simulink model "LoneWolfSimulator"  (R2023b)
settings: Solver=VariableStepAuto  StartTime=0.0  StopTime=Inf  FixedStep=0.0001  RelTol=1e-6  AbsTol=1e-6
model workspace (MAT data in the model file):
  SL_ROS_VariableLengthArrays_MaxSizes.CommonInfo.ArrayTruncateAction = 'EmitWarning'
  SL_ROS_VariableLengthArrays_MaxSizes.MsgTypeMap = containers.Map
  SL_ROS_VariableLengthArrays_MaxSizes.MsgTypeMap.serialization.keys = {'std_msgs/Float64MultiArray'}
  SL_ROS_VariableLengthArrays_MaxSizes.MsgTypeMap.serialization.values{1}.PropertyName = 'data'
  SL_ROS_VariableLengthArrays_MaxSizes.MsgTypeMap.serialization.values{1}.DataType = 'double'
  SL_ROS_VariableLengthArrays_MaxSizes.MsgTypeMap.serialization.values{1}.MaxLength = 781
  SL_ROS_VariableLengthArrays_MaxSizes.MsgTypeMap.serialization.uniformity = 0
  SL_ROS_VariableLengthArrays_MaxSizes.MsgTypeMap.serialization.keyType = 'char'
  SL_ROS_VariableLengthArrays_MaxSizes.MsgTypeMap.serialization.valueType = 'any'
values from neighbouring files (symbols this model uses):
  alpha_peak = 0.18    [LoneWolfParams.m]
  Bc = 10    [LoneWolfParams.m]
  Bl = 10    [LoneWolfParams.m]
  Cc = 1.9    [LoneWolfParams.m]
  Cl = 1.9    [LoneWolfParams.m]
  Dc = 1*g*m/2    (= 1839.375)    [LoneWolfParams.m]
  Dl = 1*g*m/2    (= 1839.375)    [LoneWolfParams.m]
  Ec = 0.97    [LoneWolfParams.m]
  El = 0.97    [LoneWolfParams.m]
  Iw = 0.5    [LoneWolfParams.m]
  Iz = (1/12) * m * (width^2 + len^2)    (= 225.015625)    [LoneWolfParams.m]
  kappa_peak = 0.18    [LoneWolfParams.m]
  m = 375    [LoneWolfParams.m]
  RRC = 5    [LoneWolfParams.m]
  wheelRadius = 0.33    [LoneWolfParams.m]
  xdotinit = 1e-3    (= 0.001)    [LoneWolfParams.m]
undefined symbols (not defined in the file or in its folder): latitude, longitude
libraries: ros2lib x11, sldrtlib x1
settings Model: Creator=bakke  LastModifiedBy=lonewolf
settings SolverCC: AutoScaleAbsTol=off  EnableFixedStepZeroCrossing=on  MaxZcBracketingIterations=100
settings OptimizationCC: EnhancedBackFolding=on  PassReuseOutputArgsAs=Individual arguments  ZeroExternalMemoryAtStartup=off  ZeroInternalMemoryAtStartup=off  MaxStackSize=64  OptimizeBlockOrder=speed  DifferentSizesBufferReuse=on  EfficientTunableParamExpr=on
settings DebuggingCC: ParameterTunabilityLossMsg=error
settings HardwareCC: ProdBitPerLong=64  ProdHWDeviceType=Intel->x86-64 (Linux 64)  UseEmbeddedCoderFeatures=off
settings RTWCC: Description=Embedded Coder  SystemTargetFile=ert.tlc  HardwareBoard=Robot Operating System 2 (ROS 2)  TLCOptions="-aInlineSetEventsForThisBaseRateFcn=TLC_FALSE -aSuppressMultiTaskScheduler=TLC_FALSE  -aRateBasedStepFcn=0"  TemplateMakefile=ert_default_tmf  Toolchain=Colcon Tools  TargetLang=C++
settings CodeAppCC: ForceParamTrailComments=on  IgnoreCustomStorageClasses=off  OperatorAnnotations=on  SimulinkDataObjDesc=on  SFDataObjDesc=on  InsertBlockDesc=on
settings ERTTargetCC: CodeInterfacePackaging=C++ class  SupportNonInlinedSFcns=on  RootIOFormat=Structure reference

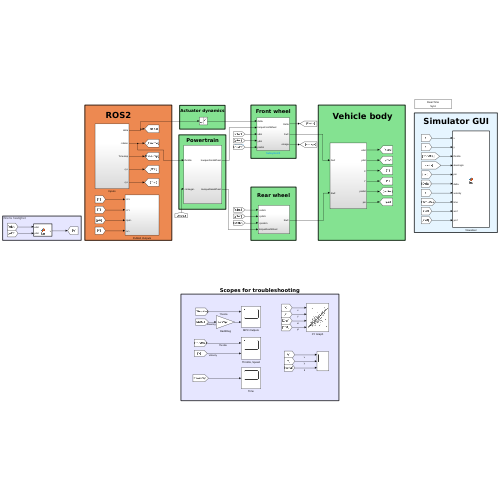
[thumbnail: Simulink's stored preview of the top-level diagram]
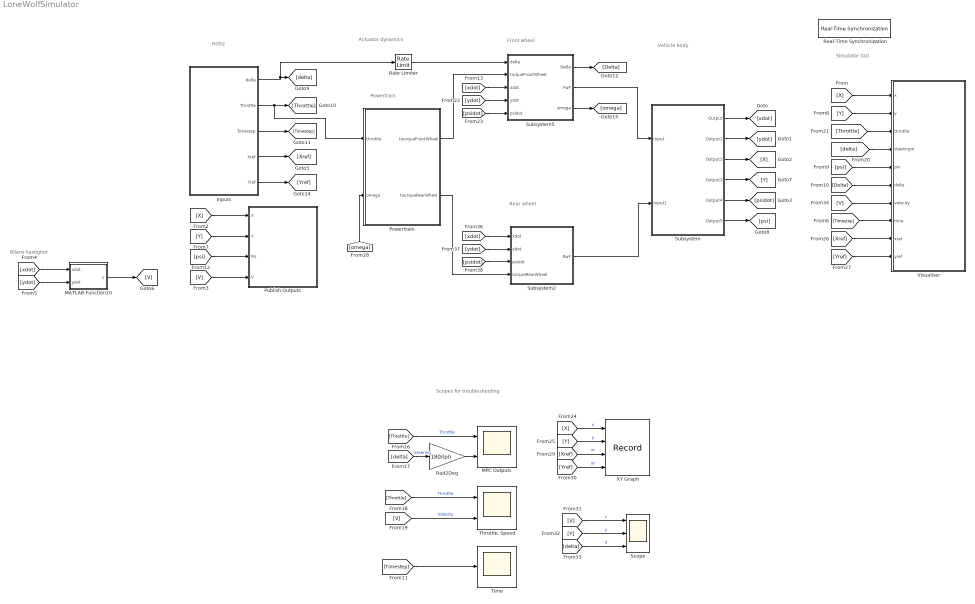
== system LoneWolfSimulator ==
  note: ROS2
  note: Bilens hastighet
  note: Simulator GUI
  note: Vehicle body
  note: Front wheel
  note: Rear wheel
  note: Powertrain
  note: Actuator dynamics
  note: Scopes for troubleshooting
  Inputs : Subsystem
  MATLAB Function10 : MATLAB Function  TreatAsAtomicUnit=on
  MPC Outputs : Scope  NumInputPorts=2
  Powertrain : Subsystem
  Publish Outputs : Subsystem
  Rad2Deg : Gain  Gain=180/(pi)
  Rate Limiter : RateLimiter  RisingSlewLimit=pi/2  FallingSlewLimit=-pi/2
  Real-Time Synchronization : sldrtlib/Real-Time Synchronization  SampleTime=0.1  MaxMissedTicks=1000  ShowMissedTicks=off  YieldWhenWaiting=off
  Scope : Scope  NumInputPorts=3
  Subsystem : Subsystem
  Subsystem2 : Subsystem
  Subsystem5 : Subsystem
  "Throttle, Speed" : Scope  NumInputPorts=2
  Time : Scope
  Visualiser : MATLAB Function  TreatAsAtomicUnit=on
  XY Graph : Record  FileSettingsInternal="{\"entries\":[{\"content\":{\"excelSettings\":{\"content\":{},\"type\":\"Streamout.ExcelSettings\"}},\"type\":\"Streamout.FileSettingStorage\",\"uuid\":\"\"}],\"packageUris\":[\"http:\\/\\/schema.mathworks.com\\/mf0\\/streamout_blocks\\/R2020a\"],\"version\":\"1.0\"}"  Layout=[1 1]  SignalsInternal="{\"entries\":[{\"content\":{\"signals\":[{\"content\":{\"blockPath\":[],\"dimensions\":[1],\"domain\":\"\",\"lineColor\":\"#edb120\",\"plots\":[ 1 ],\"port\":1,\"sid\":[\"\"],\"signalID\":1,\"signalName\":\"x\"},\"type\":\"RecordBlkView.Signal\",\"uuid\":\"\"},{\"content\":{\"blockPath\":[],\"dimensions\":[1],\"domain\":\"\",\"lineColor\":\"#7e2f8e\",\"plots\":[ 1 ],\"port\":2,\"sid\":[\"\"],\"signalID\":2,\"signalName\":\"y\"},\"type\":\"RecordBlkView.Signal\",\"uuid\":\"\"},{\"content\":{\"blockPath\":[],\"dimensions\":[1],\"domain\":\"\",\"lineColor\":\"#77ac30\",\"plots\":[ 1 ],\"port\":3,\"sid\":[\"\"],\"signalID\":3,\"signalName\":\"xr\"},\"type\":\"RecordBlkView.Signal\",\"uuid\":\"\"},{\"content\":{\"blockPath\":[],\"dimensions\":[1],\"domain\":\"\",\"lineColor\":\"#4dbeee\",\"plots\":[ 1 ],\"port\":4,\"sid\":[\"\"],\"signalID\":4,\"signalName\":\"yr\"},\"type\":\"RecordBlkView.Signal\",\"uuid\":\"\"}]},\"type\":\"RecordBlkView.InputSignals\",\"uuid\":\"\"}],\"packageUris\":[\"http:\\/\\/schema.mathworks.com\\/mf0\\/streamout_blocks\\/R2020a\"],\"version\":\"1.0\"}"  VisualizationBindings="{\"xyplotplugin\":{\"info\":[{\"series\":[{\"bindingParametersList\":[{\"parameter\":\"X-Axis\",\"signalID\":1,\"signalName\":\"x\"},{\"parameter\":\"Y-Axis\",\"signalID\":2,\"signalName\":\"y\"}],\"seriesID\":0},{\"bindingParametersList\":[{\"parameter\":\"X-Axis\",\"signalID\":3,\"signalName\":\"xr\"},{\"parameter\":\"Y-Axis\",\"signalID\":4,\"signalName\":\"yr\"}],\"seriesID\":1}],\"subplotID\":1}]}}"  CompatibilityTag=XY
  wires:
  MATLAB Function10/1(v) -> [V]
  [ydot] -> MATLAB Function10/2(ydot)
  Subsystem/1(Output) -> [xdot]
  [xdot] -> MATLAB Function10/1(xdot)
  Subsystem/2(Output1) -> [ydot]
  Subsystem/5(Output4) -> [psidot]
  Subsystem/4(Output3) -> [Y]
  Subsystem/3(Output2) -> [X]
  Subsystem/6(Output5) -> [psi]
  [X] -> Publish Outputs/1(X)
  [Y] -> Publish Outputs/2(Y)
  [psi] -> Publish Outputs/3(Psi)
  [V] -> Publish Outputs/4(V)
  [Throttle] -> MPC Outputs/1  "Throttle"
  [delta] -> Rad2Deg/1  "Steering"
  [Throttle] -> "Throttle, Speed"/1  "Throttle"
  Rad2Deg/1 -> MPC Outputs/2
  Inputs/3(Timestep) -> [Timestep]
  Inputs/4(Xref) -> [Xref]
  Inputs/5(Yref) -> [Yref]
  [omega] -> Powertrain/2(omega)
  [Timestep] -> Time/1
  [V] -> "Throttle, Speed"/2  "Velocity"
  [X] -> XY Graph/1  "x"
  [Y] -> XY Graph/2  "y"
  [Xref] -> XY Graph/3  "xr"
  [Yref] -> XY Graph/4  "yr"
  [V] -> Scope/1  "v"
  [Y] -> Scope/2  "y"
  [delta] -> Scope/3  "d"
  [V] -> Visualiser/7(velocity)
  [Delta] -> Visualiser/6(delta)
  [psi] -> Visualiser/5(psi)
  [delta] -> Visualiser/4(steeringin)
  [Throttle] -> Visualiser/3(throttle)
  [Y] -> Visualiser/2(y)
  [X] -> Visualiser/1(x)
  [Xref] -> Visualiser/9(xref)
  [Timestep] -> Visualiser/8(time)
  [Yref] -> Visualiser/10(yref)
  Powertrain/1(tourqueFrontWheel) -> Subsystem5/2(torqueFrontWheel)
  Subsystem5/1(Delta) -> [Delta]
  Subsystem5/2(FwF) -> Subsystem/1(Input)
  Subsystem5/3(omega) -> [omega]
  Powertrain/2(tourqueRearWheel) -> Subsystem2/4(torqueRearWheel)
  Subsystem2/1(RwF) -> Subsystem/2(Input1)
  Inputs/1(delta) -> [delta], Rate Limiter/1
  Inputs/2(Throttle) -> Powertrain/1(throttle), [Throttle]
  [xdot] -> Subsystem5/3(xdot)
  [ydot] -> Subsystem5/4(ydot)
  [psidot] -> Subsystem5/5(psidot)
  [xdot] -> Subsystem2/1(xdot)
  [ydot] -> Subsystem2/2(ydot)
  [psidot] -> Subsystem2/3(psidot)
  Rate Limiter/1 -> Subsystem5/1(delta)

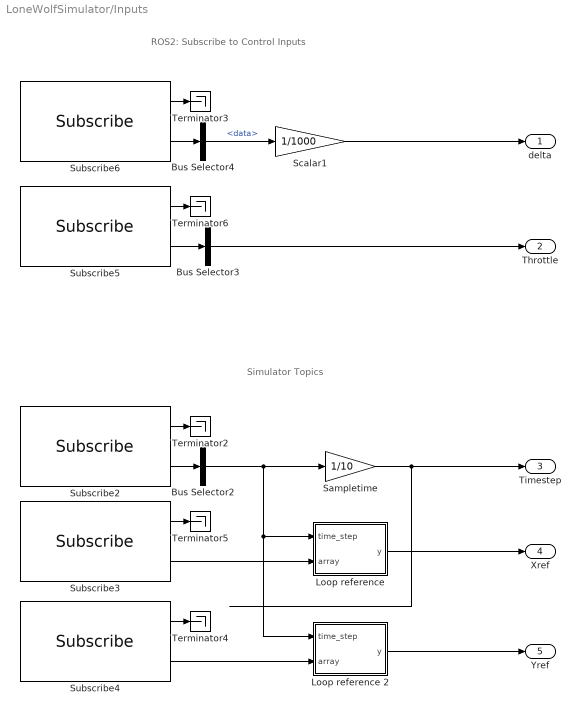
== system LoneWolfSimulator/Inputs ==
  note: ROS2: Subscribe to Control Inputs
  note: Simulator Topics
  Bus Selector2 : BusSelector  OutputSignals=data  OutputAsBus=on
  Bus Selector3 : BusSelector  OutputSignals=data  OutputAsBus=on
  Bus Selector4 : BusSelector  OutputSignals=data
  Loop reference : MATLAB Function  TreatAsAtomicUnit=on
  "Loop reference 2 " : MATLAB Function  TreatAsAtomicUnit=on
  Sampletime : Gain  Gain=1/10
  Scalar1 : Gain  Gain=1/1000
  Subscribe2 : ros2lib/Subscribe  topicSource=Specify your own  topic=/timestep  messageType=std_msgs/Int64  sampleTime=0.1  QOSHistory=Keep last  QOSDepth=1  QOSReliability=Reliable  QOSDurability=Volatile
  Subscribe3 : ros2lib/Subscribe  topicSource=Specify your own  topic=/xref  messageType=std_msgs/Float64MultiArray  sampleTime=0.1  QOSHistory=Keep last  QOSDepth=1  QOSReliability=Reliable  QOSDurability=Volatile
  Subscribe4 : ros2lib/Subscribe  topicSource=Specify your own  topic=/yref  messageType=std_msgs/Float64MultiArray  sampleTime=0.1  QOSHistory=Keep last  QOSDepth=1  QOSReliability=Reliable  QOSDurability=Volatile
  Subscribe5 : ros2lib/Subscribe  topicSource=Specify your own  topic=/lw_portenta_throttle  messageType=std_msgs/Int64  sampleTime=0.1  QOSHistory=Keep last  QOSDepth=1  QOSReliability=Reliable  QOSDurability=Volatile
  Subscribe6 : ros2lib/Subscribe  topicSource=Specify your own  topic=/lw_portenta_steering  messageType=std_msgs/Int64  sampleTime=0.1  QOSHistory=Keep last  QOSDepth=1  QOSReliability=Reliable  QOSDurability=Volatile
  Terminator{2..6} (5 alike) : Terminator
  delta : Outport
  Throttle : Outport  Port=2
  Timestep : Outport  Port=3
  Xref : Outport  Port=4
  Yref : Outport  Port=5
  wires:
  Subscribe2/1 -> Terminator2/1
  Subscribe2/2 -> Bus Selector2/1
  Sampletime/1 -> Timestep/1
  Subscribe4/1 -> Terminator4/1
  Subscribe4/2 -> "Loop reference 2 "/2(array)
  Subscribe3/2 -> Loop reference/2(array)
  Subscribe3/1 -> Terminator5/1
  Loop reference/1(y) -> Xref/1
  "Loop reference 2 "/1(y) -> Yref/1
  Bus Selector2/1 -> Sampletime/1, "Loop reference 2 "/1(time_step), Loop reference/1(time_step)
  Subscribe5/2 -> Bus Selector3/1
  Scalar1/1 -> delta/1
  Bus Selector3/1 -> Throttle/1
  Subscribe6/1 -> Terminator3/1
  Subscribe5/1 -> Terminator6/1
  Subscribe6/2 -> Bus Selector4/1
  Bus Selector4/1 -> Scalar1/1  "<data>"

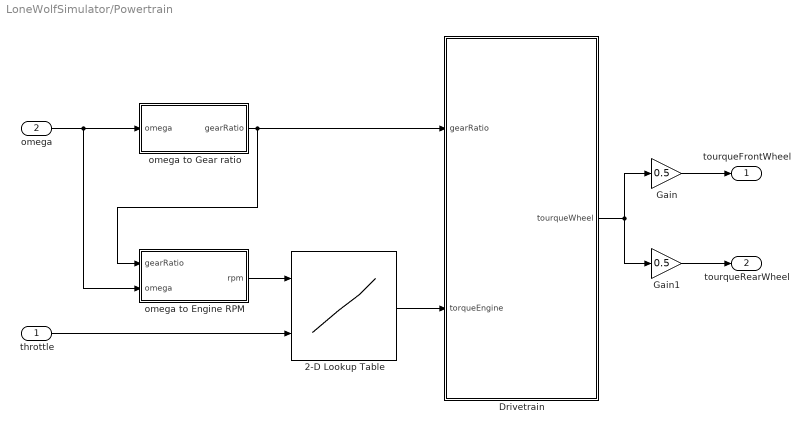
== system LoneWolfSimulator/Powertrain ==
  throttle : Inport
  omega : Inport  Port=2
  2-D Lookup Table : Lookup_n-D  BreakpointsForDimension1=[0;169.614855264094;367.085957899886;589.246670617181;789.821522752712;996.567251474744;1181.71186027627;1425.48895225281;1626.06685625609;1835.92854194885;2042.68342627413;2243.26743401291;2425.36017506641;2616.68481605769;2860.48021924071;3085.77825200297;3264.76724355674;3468.45194892751;3656.70641096427;3909.77338836579;4131.97377536381;4314.05736081407;4493.04635236784;4696.71885026762;4909.65376678264;5110.24998199241;5292.32135997168;5499.07014056146;5718.17288179523;5965.03541206502;6199.56534476505;6390.87472641759;6582.16884873138;6758.05409078541;6980.20259603171]  BreakpointsForDimension2=[0;10;20;30;40;50;60;70;80;90;100]  Table=[0.3 7.52683562951347 11.8387627553835 13.7538912505429 14.2370681748395 17.110514311951 18.5474885119643 17.5896731329271 18.0683296909882 19.0271495958556 24.298398889508;0.2 10.3686392029757 12.7749808290727 17.5615464096832 19.4852133743988 21.8820120051095 25.2300965969615 24.7539513534759 28.0985201049223 31.4546409034155 33.8484259566359;0 11.2978255958539 15.1431504736246 22.3255101591157 25.2084992916136 29.038254019017 37.6505562237105 34.7881598707304 46.2688855833847 47.2272032253369 51.5386280882919;0 13.1858318935994 20.8624182875188 30.4380607633152 37.1492978344714 39.5491100426724 54.8631063231358 53.915838465315 65.4061071733557 67.8013990153211 73.0706392573133;0 16.0346671478725 30.4094317771563 43.3462176805965 52.4527465937181 63.4723949503387 69.6994505713682 77.3680007586463 84.553876284543 88.8678124620733 88.8688169879034;-2.44629412790408 24.6344127796893 47.1563841543122 73.0294536982776 73.0379921678338 91.720665819667 102.743327753778 118.552053005585 116.160277004025 127.660088707451 124.308990538109;-4.96800884998436 35.1502914324955 71.0816781136389 103.177785175313 114.222546677687 132.430079611865 148.722986313798 180.336920977006 188.48362545943 193.279734035427 163.107293938468;-8.74578514092923 33.6856927721534 72.4880142758329 104.587637177913 130.961462848202 155.87470796147 177.437859431226 195.635347107102 209.529446126664 221.029760093006 226.319090851601;-12.1015317204333 33.6520411568438 75.3288133234649 113.858360154898 143.370370427905 164.462399283325 190.810609544946 214.287382721116 229.13779033097 243.993220569975 247.83502960734;-19.201920026761 35.0558660044625 81.0551128181702 121.980453754484 158.198176206581 185.034586021649 211.865973207567 232.947956804686 250.676330917887 265.053104598831 277.032075123234;-23.3903905203684 35.0282415441337 84.3810978417591 127.227594428213 165.359943112554 196.510289105152 225.735461344291 249.691393341436 267.899930801444 284.190326188802 296.649460060012;-27.5779890517621 31.4144554912304 86.2680996136746 133.424012011423 173.479023134649 206.067347853091 234.811352219593 263.073686450543 283.200365983201 296.143179041622 314.343680294988;-34.6744535281279 28.5083622646395 84.8029986904173 132.424508810435 174.403689161292 210.348636941142 239.083600575173 265.9119741836 288.438465924458 303.782095716911 318.144303773318;-38.4448181402563 22.7303296896822 79.0219525379695 127.60881198075 170.065644363838 207.922707061357 236.655159380812 261.571418071571 285.059241031872 302.791633248394 315.243735438792;-44.7181502868699 19.3501002712657 76.5965249210998 125.188909255946 170.034504063104 205.489745500762 237.114227685186 262.989306280812 284.552457750567 303.239651768636 317.613914135005;-53.0684964265662 14.5328966528359 72.7336208413018 123.725817384349 168.093257896361 204.501292083905 235.646615447353 263.444356481864 285.961807490252 304.168335898599 318.061932655246;-57.6689690661566 10.1943495924673 67.9169194857871 119.863917830381 165.197712190987 201.122569454234 232.254331718975 261.012399447099 284.010516065207 301.740396967154 318.513467015894;-63.9366334583809 4.41481022876471 62.1353710704242 114.762859997277 162.775298151607 195.485378400082 228.870586460153 255.707498538137 277.747799777208 296.440518687343 312.256777882875;-69.7861919691262 -2.32304677689018 58.7496167599421 109.939629223867 157.474917608881 193.058946257382 225.968009073968 255.203226571407 278.19581829745 296.410885175354 312.707307717692;-78.1404619387842 -9.54508523267177 53.452249794706 105.592543693942 154.556770072328 190.157373397027 224.031785536375 252.782821583688 275.782444990542 295.429463439308 311.718854300836;-84.8266681935945 -12.4471603559423 48.6390642795968 102.692979885247 151.179554231402 188.687752107534 223.0493592745 251.318725186261 274.317344067285 293.481687854669 309.292422158136;-90.6753547421262 -16.3085576469951 45.7379936821564 99.7888957103159 147.799324812986 188.655607280969 222.54508730777 250.807923801635 ...(+2434 chars)]  InternalRulePriority=Speed  RndMeth=Simplest
      settings: InputPortMap=u0,u1
  Drivetrain : MATLAB Function  TreatAsAtomicUnit=on
  Gain : Gain  Gain=0.5
  Gain1 : Gain  Gain=0.5
  omega to Engine RPM : MATLAB Function  TreatAsAtomicUnit=on
  omega to Gear ratio : MATLAB Function  TreatAsAtomicUnit=on
  tourqueFrontWheel : Outport
  tourqueRearWheel : Outport  Port=2
  wires:
  omega to Gear ratio/1(gearRatio) -> omega to Engine RPM/1(gearRatio), Drivetrain/1(gearRatio)
  2-D Lookup Table/1 -> Drivetrain/2(torqueEngine)
  throttle/1 -> 2-D Lookup Table/2
  omega/1 -> omega to Gear ratio/1(omega), omega to Engine RPM/2(omega)
  omega to Engine RPM/1(rpm) -> 2-D Lookup Table/1
  Drivetrain/1(tourqueWheel) -> Gain1/1, Gain/1
  Gain/1 -> tourqueFrontWheel/1
  Gain1/1 -> tourqueRearWheel/1

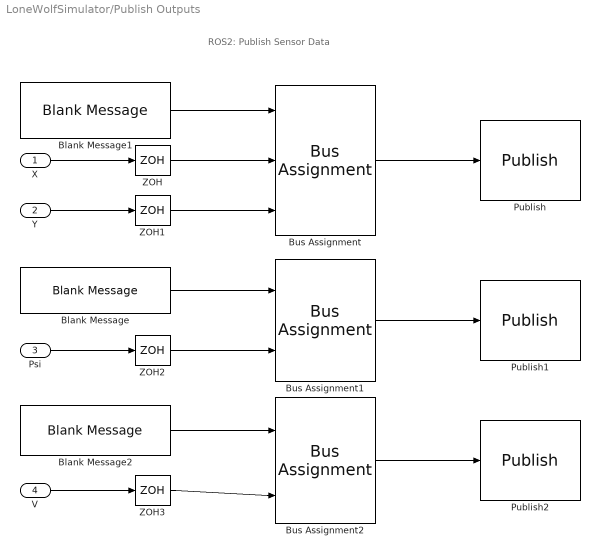
== system LoneWolfSimulator/Publish Outputs ==
  note: ROS2: Publish Sensor Data
  X : Inport
  Y : Inport  Port=2
  Psi : Inport  Port=3
  V : Inport  Port=4
  Blank Message : ros2lib/Blank Message  messageClass=Message  entityType=geometry_msgs/PoseWithCovarianceStamped  messageType=geometry_msgs/PoseWithCovarianceStamped  SampleTime=0.1
  Blank Message1 : ros2lib/Blank Message  messageClass=Message  entityType=sensor_msgs/NavSatFix  messageType=sensor_msgs/NavSatFix  SampleTime=0.1
  Blank Message2 : ros2lib/Blank Message  messageClass=Message  entityType=geometry_msgs/TwistWithCovarianceStamped  messageType=geometry_msgs/TwistWithCovarianceStamped  SampleTime=0.1
  Bus Assignment : BusAssignment  AssignedSignals=latitude,longitude
  Bus Assignment1 : BusAssignment  AssignedSignals=pose.pose.position.z
  Bus Assignment2 : BusAssignment  AssignedSignals=twist.twist.linear.x
  Publish : ros2lib/Publish  topicSource=Specify your own  topic=/vectornav/gnss  messageType=sensor_msgs/NavSatFix  QOSHistory=Keep last  QOSDepth=1  QOSReliability=Reliable  QOSDurability=Volatile
  Publish1 : ros2lib/Publish  topicSource=Specify your own  topic=/vectornav/pose  messageType=geometry_msgs/PoseWithCovarianceStamped  QOSHistory=Keep last  QOSDepth=1  QOSReliability=Reliable  QOSDurability=Volatile
  Publish2 : ros2lib/Publish  topicSource=Specify your own  topic=/vectornav/velocity_body  messageType=geometry_msgs/TwistWithCovarianceStamped  QOSHistory=Keep last  QOSDepth=1  QOSReliability=Reliable  QOSDurability=Volatile
  ZOH{,1..3} (4 alike) : ZeroOrderHold  SampleTime=0.1
  wires:
  Blank Message/1 -> Bus Assignment1/1
  Bus Assignment1/1 -> Publish1/1
  ZOH3/1 -> Bus Assignment2/2
  Bus Assignment2/1 -> Publish2/1
  ZOH2/1 -> Bus Assignment1/2
  Psi/1 -> ZOH2/1
  Blank Message1/1 -> Bus Assignment/1
  V/1 -> ZOH3/1
  X/1 -> ZOH/1
  ZOH/1 -> Bus Assignment/2
  Bus Assignment/1 -> Publish/1
  Blank Message2/1 -> Bus Assignment2/1
  Y/1 -> ZOH1/1
  ZOH1/1 -> Bus Assignment/3

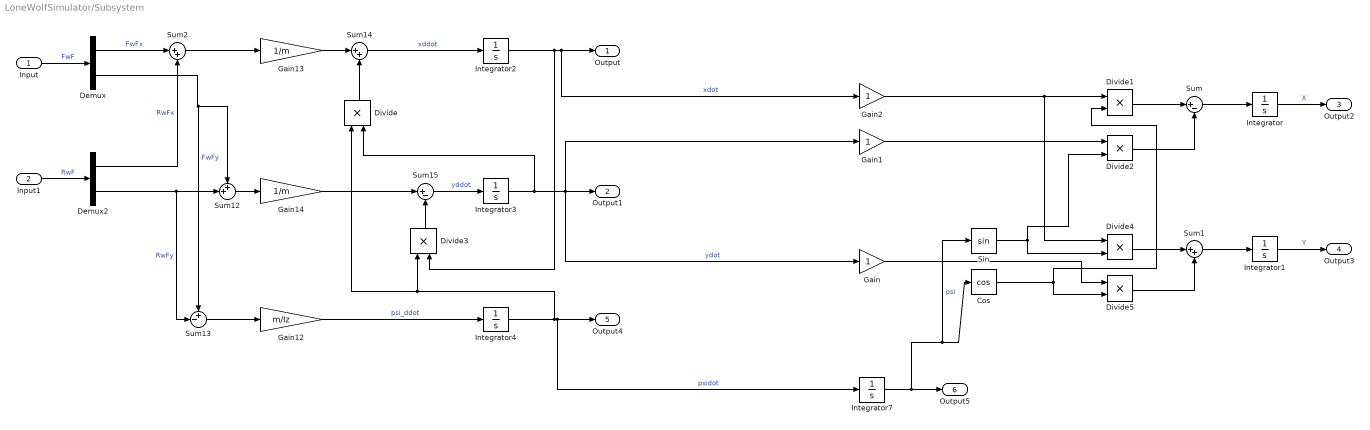
== system LoneWolfSimulator/Subsystem ==
  Input : Inport
  Input1 : Inport  Port=2
  Cos : Trigonometry  Operator=cos
  Demux : Demux  Outputs=2
  Demux2 : Demux  Outputs=2
  Divide{,1..5} (6 alike) : Product  Inputs=**
  Gain : Gain
  Gain1 : Gain
  Gain12 : Gain  Gain=m/Iz
  Gain13 : Gain  Gain=1/m
  Gain14 : Gain  Gain=1/m
  Gain2 : Gain
  Integrator{,1,3..4,7} (5 alike) : Integrator
  Integrator2 : Integrator  InitialCondition=xdotinit
  Sin : Trigonometry
  Sum : Sum  Inputs=|+-
  Sum1 : Sum  Inputs=|++
  Sum12 : Sum  Inputs=++|
  Sum13 : Sum  Inputs=+-|
  Sum14 : Sum  Inputs=|++
  Sum15 : Sum  Inputs=|+-
  Sum2 : Sum  Inputs=|++
  Output : Outport
  Output1 : Outport  Port=2
  Output2 : Outport  Port=3
  Output3 : Outport  Port=4
  Output4 : Outport  Port=5
  Output5 : Outport  Port=6
  wires:
  Demux2/1 -> Sum2/2  "RwFx"
  Input/1 -> Demux/1  "FwF"
  Demux/1 -> Sum2/1  "FwFx"
  Demux2/2 -> Sum12/2, Sum13/2  "RwFy"
  Integrator2/1 -> Gain2/1, Output/1, Divide3/2  "xdot"
  Sum13/1 -> Gain12/1
  Integrator4/1 -> Integrator7/1, Output4/1, Divide/1, Divide3/1  "psidot"
  Sum14/1 -> Integrator2/1  "xddot"
  Demux/2 -> Sum12/1, Sum13/1  "FwFy"
  Input1/1 -> Demux2/1  "RwF"
  Gain13/1 -> Sum14/1
  Integrator7/1 -> Output5/1, Cos/1, Sin/1  "psi"
  Gain14/1 -> Sum15/1
  Integrator3/1 -> Gain1/1, Gain/1, Output1/1, Divide/2  "ydot"
  Divide3/1 -> Sum15/2
  Gain12/1 -> Integrator4/1  "psi_ddot"
  Sum2/1 -> Gain13/1
  Sum15/1 -> Integrator3/1  "yddot"
  Sum12/1 -> Gain14/1
  Divide/1 -> Sum14/2
  Cos/1 -> Divide5/2, Divide1/2
  Sin/1 -> Divide4/2, Divide2/2
  Divide1/1 -> Sum/1
  Divide2/1 -> Sum/2
  Divide4/1 -> Sum1/1
  Divide5/1 -> Sum1/2
  Sum/1 -> Integrator/1
  Integrator/1 -> Output2/1  "X"
  Sum1/1 -> Integrator1/1
  Integrator1/1 -> Output3/1  "Y"
  Gain/1 -> Divide5/1
  Gain1/1 -> Divide2/1
  Gain2/1 -> Divide1/1, Divide4/1

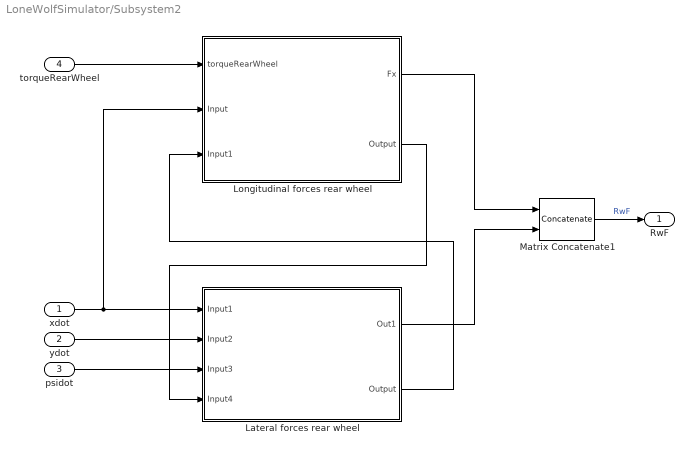
== system LoneWolfSimulator/Subsystem2 ==
  xdot : Inport
  ydot : Inport  Port=2
  psidot : Inport  Port=3
  torqueRearWheel : Inport  Port=4
  Lateral forces rear wheel : Subsystem
  Longitudinal forces rear wheel : Subsystem
  Matrix Concatenate1 : Concatenate  Mode=Multidimensional array
  RwF : Outport
  wires:
  Longitudinal forces rear wheel/2(Output) -> Lateral forces rear wheel/4(Input4)
  Lateral forces rear wheel/2(Output) -> Longitudinal forces rear wheel/3(Input1)
  torqueRearWheel/1 -> Longitudinal forces rear wheel/1(torqueRearWheel)
  xdot/1 -> Lateral forces rear wheel/1(Input1), Longitudinal forces rear wheel/2(Input)
  ydot/1 -> Lateral forces rear wheel/2(Input2)
  psidot/1 -> Lateral forces rear wheel/3(Input3)
  Lateral forces rear wheel/1(Out1) -> Matrix Concatenate1/2
  Longitudinal forces rear wheel/1(Fx) -> Matrix Concatenate1/1
  Matrix Concatenate1/1 -> RwF/1  "RwF"

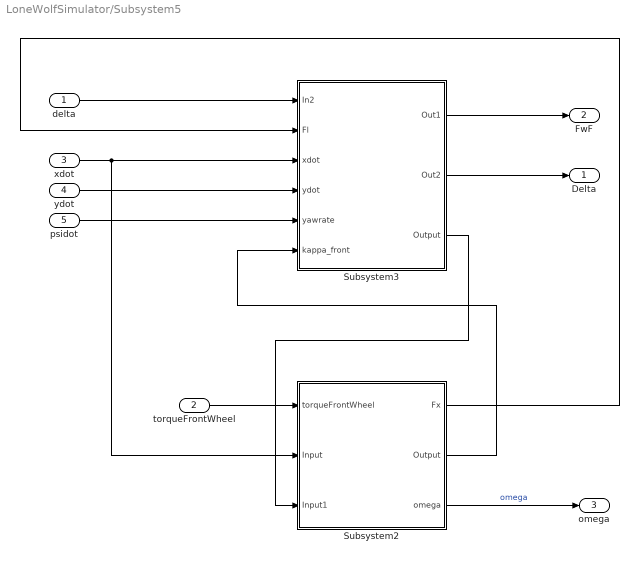
== system LoneWolfSimulator/Subsystem5 ==
  delta : Inport
  torqueFrontWheel : Inport  Port=2
  xdot : Inport  Port=3
  ydot : Inport  Port=4
  psidot : Inport  Port=5
  Subsystem2 : Subsystem
  Subsystem3 : Subsystem
  Delta : Outport
  FwF : Outport  Port=2
  omega : Outport  Port=3
  wires:
  Subsystem2/2(Output) -> Subsystem3/6(kappa_front)
  Subsystem3/2(Out2) -> Delta/1
  Subsystem3/1(Out1) -> FwF/1
  ydot/1 -> Subsystem3/4(ydot)
  psidot/1 -> Subsystem3/5(yawrate)
  Subsystem2/3(omega) -> omega/1  "omega"
  xdot/1 -> Subsystem2/2(Input), Subsystem3/3(xdot)
  torqueFrontWheel/1 -> Subsystem2/1(torqueFrontWheel)
  delta/1 -> Subsystem3/1(In2)
  Subsystem3/3(Output) -> Subsystem2/3(Input1)
  Subsystem2/1(Fx) -> Subsystem3/2(Fl)

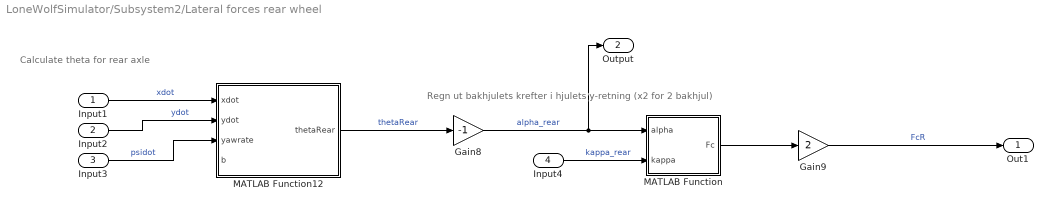
== system LoneWolfSimulator/Subsystem2/Lateral forces rear wheel ==
  note: Regn ut bakhjulets krefter i hjulets y-retning (x2 for 2 bakhjul)
  note: Calculate theta for rear axle
  Input1 : Inport
  Input2 : Inport  Port=2
  Input3 : Inport  Port=3
  Input4 : Inport  Port=4
  Gain8 : Gain  Gain=-1
  Gain9 : Gain  Gain=2
  MATLAB Function : MATLAB Function  TreatAsAtomicUnit=on
  MATLAB Function12 : MATLAB Function  TreatAsAtomicUnit=on
  Out1 : Outport
  Output : Outport  Port=2
  wires:
  Gain9/1 -> Out1/1  "FcR"
  Gain8/1 -> MATLAB Function/1(alpha), Output/1  "alpha_rear"
  MATLAB Function12/1(thetaRear) -> Gain8/1  "thetaRear"
  Input3/1 -> MATLAB Function12/3(yawrate)  "psidot"
  Input2/1 -> MATLAB Function12/2(ydot)  "ydot"
  Input1/1 -> MATLAB Function12/1(xdot)  "xdot"
  MATLAB Function/1(Fc) -> Gain9/1
  Input4/1 -> MATLAB Function/2(kappa)  "kappa_rear"

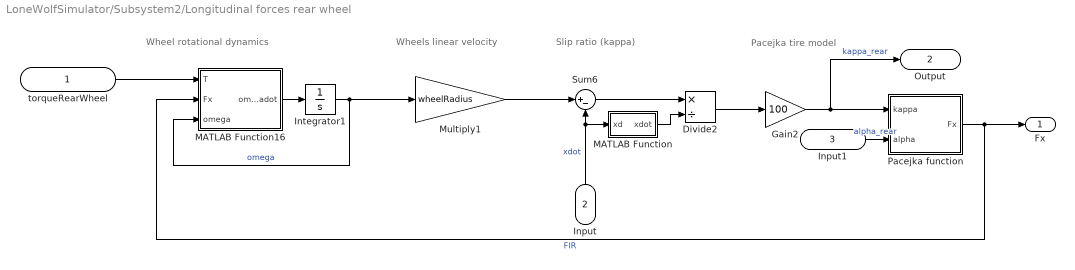
== system LoneWolfSimulator/Subsystem2/Longitudinal forces rear wheel ==
  note: Pacejka tire model
  note: Slip ratio (kappa)
  note: Wheels linear velocity
  note: Wheel rotational dynamics
  torqueRearWheel : Inport
  Input : Inport  Port=2
  Input1 : Inport  Port=3
  Divide2 : Product  Inputs=*/
  Gain2 : Gain  Gain=100
  Integrator1 : Integrator  InitialCondition=(xdotinit)/0.3
  MATLAB Function : MATLAB Function  TreatAsAtomicUnit=on
  MATLAB Function16 : MATLAB Function  TreatAsAtomicUnit=on
  Multiply1 : Gain  Gain=wheelRadius
  Pacejka function : MATLAB Function  TreatAsAtomicUnit=on
  Sum6 : Sum  Inputs=|+-
  Fx : Outport
  Output : Outport  Port=2
  wires:
  Pacejka function/1(Fx) -> Fx/1, MATLAB Function16/2(Fx)  "FlR"
  Divide2/1 -> Gain2/1
  MATLAB Function16/1(omegadot) -> Integrator1/1
  Integrator1/1 -> Multiply1/1, MATLAB Function16/3(omega)  "omega"
  Multiply1/1 -> Sum6/1
  Sum6/1 -> Divide2/1
  Input/1 -> Sum6/2, MATLAB Function/1(xd)  "xdot"
  MATLAB Function/1(xdot) -> Divide2/2
  Gain2/1 -> Pacejka function/1(kappa), Output/1  "kappa_rear"
  torqueRearWheel/1 -> MATLAB Function16/1(T)
  Input1/1 -> Pacejka function/2(alpha)  "alpha_rear"

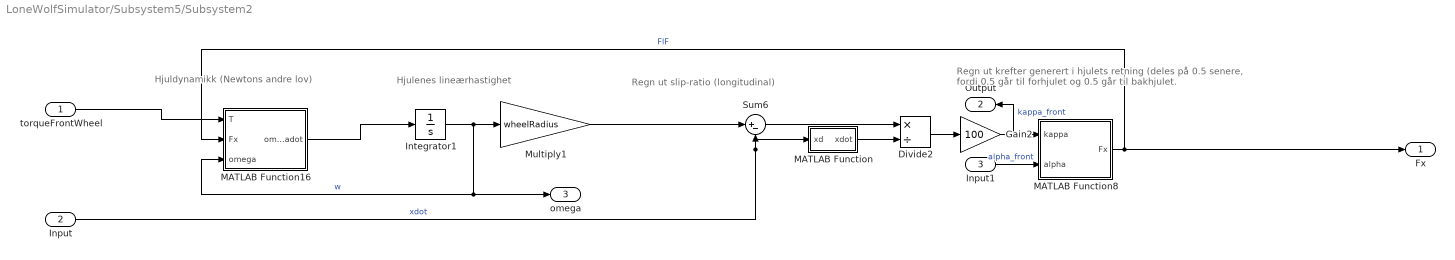
== system LoneWolfSimulator/Subsystem5/Subsystem2 ==
  note: Hjulenes lineærhastighet
  note: Regn ut krefter generert i hjulets retning (deles på 0.5 senere, fordi 0.5 går til forhjulet og 0.5 går til bakhjulet.
  note: Regn ut slip-ratio (longitudinal)
  note: Hjuldynamikk (Newtons andre lov)
  torqueFrontWheel : Inport
  Input : Inport  Port=2
  Input1 : Inport  Port=3
  Divide2 : Product  Inputs=*/
  Gain2 : Gain  Gain=100
  Integrator1 : Integrator  InitialCondition=(xdotinit)/0.3
  MATLAB Function : MATLAB Function  TreatAsAtomicUnit=on
  MATLAB Function16 : MATLAB Function  TreatAsAtomicUnit=on
  MATLAB Function8 : MATLAB Function  TreatAsAtomicUnit=on
  Multiply1 : Gain  Gain=wheelRadius
  Sum6 : Sum  Inputs=|+-
  Fx : Outport
  Output : Outport  Port=2
  omega : Outport  Port=3
  wires:
  MATLAB Function8/1(Fx) -> Fx/1, MATLAB Function16/2(Fx)  "FlF"
  Divide2/1 -> Gain2/1
  MATLAB Function16/1(omegadot) -> Integrator1/1
  Integrator1/1 -> Multiply1/1, omega/1, MATLAB Function16/3(omega)  "w"
  Multiply1/1 -> Sum6/1
  Sum6/1 -> Divide2/1
  Input/1 -> MATLAB Function/1(xd), Sum6/2  "xdot"
  MATLAB Function/1(xdot) -> Divide2/2
  Gain2/1 -> MATLAB Function8/1(kappa), Output/1  "kappa_front"
  torqueFrontWheel/1 -> MATLAB Function16/1(T)
  Input1/1 -> MATLAB Function8/2(alpha)  "alpha_front"

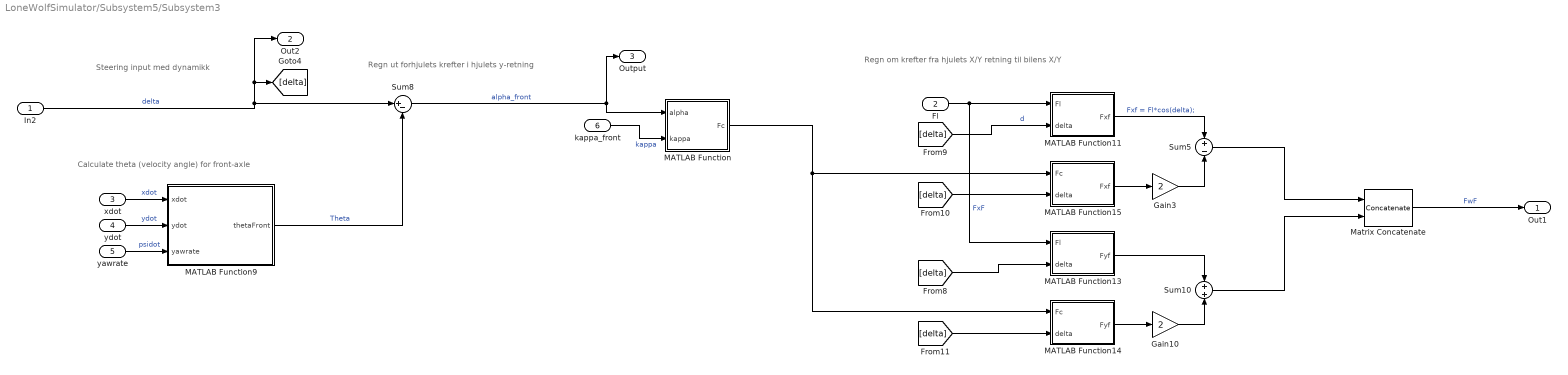
== system LoneWolfSimulator/Subsystem5/Subsystem3 ==
  note: Regn om krefter fra hjulets X/Y retning til bilens X/Y
  note: Steering input med dynamikk
  note: Regn ut forhjulets krefter i hjulets y-retning
  note: Calculate theta (velocity angle) for front-axle
  In2 : Inport
  Fl : Inport  Port=2
  xdot : Inport  Port=3
  ydot : Inport  Port=4
  yawrate : Inport  Port=5
  kappa_front : Inport  Port=6
  Gain10 : Gain  Gain=2
  Gain3 : Gain  Gain=2
  MATLAB Function : MATLAB Function  TreatAsAtomicUnit=on
  MATLAB Function11 : MATLAB Function  TreatAsAtomicUnit=on
  MATLAB Function13 : MATLAB Function  TreatAsAtomicUnit=on
  MATLAB Function14 : MATLAB Function  TreatAsAtomicUnit=on
  MATLAB Function15 : MATLAB Function  TreatAsAtomicUnit=on
  MATLAB Function9 : MATLAB Function  TreatAsAtomicUnit=on
  Matrix Concatenate : Concatenate  Mode=Multidimensional array
  Sum10 : Sum  Inputs=+|+
  Sum5 : Sum  Inputs=+|-
  Sum8 : Sum  Inputs=|+-
  Out1 : Outport
  Out2 : Outport  Port=2
  Output : Outport  Port=3
  wires:
  Gain3/1 -> Sum5/2
  Sum10/1 -> Matrix Concatenate/2
  MATLAB Function11/1(Fxf) -> Sum5/1  "Fxf = Fl*cos(delta);"
  [delta] -> MATLAB Function11/2(delta)  "d"
  MATLAB Function15/1(Fxf) -> Gain3/1
  Sum5/1 -> Matrix Concatenate/1
  [delta] -> MATLAB Function15/2(delta)
  MATLAB Function9/1(thetaFront) -> Sum8/2  "Theta"
  Gain10/1 -> Sum10/2
  [delta] -> MATLAB Function14/2(delta)
  MATLAB Function13/1(Fyf) -> Sum10/1
  Sum8/1 -> Output/1, MATLAB Function/1(alpha)  "alpha_front"
  MATLAB Function14/1(Fyf) -> Gain10/1
  [delta] -> MATLAB Function13/2(delta)
  Matrix Concatenate/1 -> Out1/1  "FwF"
  In2/1 -> [delta], Out2/1, Sum8/1  "delta"
  Fl/1 -> MATLAB Function11/1(Fl), MATLAB Function13/1(Fl)  "FxF"
  xdot/1 -> MATLAB Function9/1(xdot)  "xdot"
  ydot/1 -> MATLAB Function9/2(ydot)  "ydot"
  yawrate/1 -> MATLAB Function9/3(yawrate)  "psidot"
  MATLAB Function/1(Fc) -> MATLAB Function15/1(Fc), MATLAB Function14/1(Fc)
  kappa_front/1 -> MATLAB Function/2(kappa)  "kappa"

== matlab function LoneWolfSimulator/Subsystem5/Subsystem2/MATLAB Function8 ==
  data: Fx output; Bl parameter; Cl parameter; Dl parameter; El parameter; kappa_peak parameter; alpha_peak parameter; kappa input; alpha input
function Fx = fcn(Bl, Cl, Dl, El, kappa_peak, alpha_peak, kappa, alpha)

alpha_norm = alpha/alpha_peak;
kappa_norm = kappa/kappa_peak;

S = sqrt(alpha_norm^2+kappa_norm^2);

kappa_mod = S * alpha_peak;

Fx = kappa_norm/S * Dl*sin(Cl*atan(Bl*kappa_mod-El*(Bl*kappa_mod-atan(Bl*kappa_mod))));

== matlab function LoneWolfSimulator/Subsystem5/Subsystem3/MATLAB Function9 ==
  data: xdot input; thetaFront output; ydot input; yawrate input
function thetaFront = fcn(xdot, ydot, yawrate)

thetaFront = atan((ydot+yawrate*1.4)/xdot);

== matlab function LoneWolfSimulator/Subsystem2/Lateral forces rear wheel/MATLAB Function12 ==
  data: xdot input; thetaRear output; ydot input; yawrate input; b input
function thetaRear = fcn(xdot, ydot, yawrate, b)

thetaRear = atan((ydot-yawrate*b)/xdot);

== matlab function LoneWolfSimulator/Subsystem5/Subsystem3/MATLAB Function13 ==
  data: Fl input; Fyf output; delta input
function Fyf = fcn(Fl, delta)

Fyf = Fl*sin(delta);

== matlab function LoneWolfSimulator/Subsystem5/Subsystem3/MATLAB Function14 ==
  data: Fc input; delta input; Fyf output
function Fyf = fcn(Fc, delta)

Fyf = Fc*cos(delta);

== matlab function LoneWolfSimulator/Subsystem5/Subsystem3/MATLAB Function15 ==
  data: Fc input; Fxf output; delta input
function Fxf = fcn(Fc, delta)

Fxf = Fc*sin(delta);

== matlab function LoneWolfSimulator/Subsystem5/Subsystem2/MATLAB Function16 ==
  data: T input; omegadot output; Fx input; omega input; wheelRadius parameter; Iw parameter; RRC parameter
function omegadot = fcn(T, Fx, omega, wheelRadius, Iw, RRC)

omegadot = (T - wheelRadius * Fx - RRC * omega)/Iw;

% 0.5 = Hjulets treghetsmoment
% 8 * omega motorbrems / rullemotstand

== matlab function LoneWolfSimulator/Powertrain/omega to Engine RPM ==
  data: gearRatio input; omega input; rpm output
function rpm = fcn(gearRatio, omega)


rpm = (omega*9.55)*gearRatio*4.04;

== matlab function LoneWolfSimulator/Powertrain/omega to Gear ratio ==
  data: omega input; gearRatio output
function gearRatio = fcn(omega)

velLimitLow = 3.72;
velLimitHigh = 12;
lowRatio = 5.952;
highRatio = 3.691;
velocity = omega*0.33;

if (velocity < velLimitLow)
    gearRatio = lowRatio;
elseif (velLimitLow < velocity && velocity < velLimitHigh)
    gearRatio = lowRatio - (velocity-velLimitLow)/(velLimitHigh-velLimitLow)*2.26;
else
    gearRatio = highRatio;
end

== matlab function LoneWolfSimulator/Powertrain/Drivetrain ==
  data: gearRatio input; torqueEngine input; tourqueWheel output; FinalDrive_gear_ratio parameter
function tourqueWheel = fcn(gearRatio,torqueEngine, FinalDrive_gear_ratio)

tourqueWheel = torqueEngine*gearRatio* FinalDrive_gear_ratio*(1/8.89); % magic number shhhh scaling for 60km/h topspeed

== matlab function LoneWolfSimulator/Inputs/Loop reference ==
  data: time_step input; array input; y output
function y = fcn(time_step, array)
    % index = mod(time_step, N_STEPS_REFERENCE) + 1;
    index = mod(time_step, length(array.data)) + 1; 
    y = array.data(index);
end

== matlab function LoneWolfSimulator/Subsystem2/Lateral forces rear wheel/MATLAB Function ==
  data: alpha input; Fc output; kappa input; Bc parameter; Cc parameter; Dc parameter; Ec parameter; alpha_peak parameter; kappa_peak parameter
function Fc = fcn(alpha, kappa, Bc, Cc, Dc, Ec, alpha_peak, kappa_peak)

alpha_norm = alpha/alpha_peak;
kappa_norm = kappa/kappa_peak;

S = sqrt(alpha_norm^2+kappa_norm^2);

alpha_mod = S * alpha_peak;

Fc = alpha_norm/S * Dc*sin(Cc*atan(Bc*alpha_mod-Ec*(Bc*alpha_mod-atan(Bc*alpha_mod))));

== matlab function LoneWolfSimulator/Inputs/Loop reference 2  ==
  data: time_step input; array input; y output
function y = fcn(time_step, array)
    % index = mod(time_step, N_STEPS_REFERENCE) + 1;
    index = mod(time_step, length(array.data)) + 1; 
    y = array.data(index);
end

== matlab function LoneWolfSimulator/Visualiser ==
  settings: updateMethod=DISCRETE  sampleTime=0.1
  data: x input; y input; throttle input; steeringin input; psi input; delta input; velocity input; time input; xref input; yref input
function fnc(x, y, throttle, steeringin, psi, delta, velocity, time, xref, yref)
    persistent xmin xmax ymin ymax vehiclePathX vehiclePathY posErrorPlot errorArray refPathX refPathY vehicleFig pathPlot refPlot leftWheelPatch rightWheelPatch rearLeftWheelPatch rearRightWheelPatch lwPatch velocityPlot deltaPlot timeArray deltaArray velocityArray throttleArray steeringinArray steeringinPlot throttlePlot 
    
    lwWidth = 2.4;
    lwHeight = 1.2;
    wheelWidth = 0.66;
    wheelHeight = 0.22;

    if isempty(vehicleFig)
        vehicleFig = figure('WindowState','maximized');
        hold on;
        subplot(3,7,[1:3 8:10 15:17]);
        pathPlot = plot(NaN, NaN, 'k-', 'LineWidth', 2);
        hold on;
        refPlot = plot(NaN, NaN, 'b:', 'LineWidth', 2);
        axis equal;
        grid on;
        xlabel('X', 'FontSize', 10, 'FontName','Garamound', 'FontWeight','bold');
        ylabel('Y', 'FontSize', 10, 'FontName','Garamound', 'FontWeight','bold','Rotation',0);
        set(gca, 'FontSize', 15); % Set the font size for the tick labels
        leftWheelPatch = patch('XData', [], 'YData', [], 'FaceColor', 'k', 'EdgeColor', 'k');
        rightWheelPatch = patch('XData', [], 'YData', [], 'FaceColor', 'k', 'EdgeColor', 'k');
        rearLeftWheelPatch = patch('XData', [], 'YData', [], 'FaceColor', 'k', 'EdgeColor', 'k');
        rearRightWheelPatch = patch('XData', [], 'YData', [], 'FaceColor', 'k', 'EdgeColor', 'k');
        lwPatch = patch('XData', [], 'YData', [], 'FaceColor', 'r', 'EdgeColor', 'k');
        xmin = -15;
        xmax = 15;
        ymin = -15;
        ymax = 15;

        timeArray = [];
        velocityArray = [];
        deltaArray = [];
        errorArray = [];
        throttleArray = [];
        steeringinArray = [];

        subplot(3,7,5:7);
        velocityPlot = plot(NaN, NaN, 'g-', 'LineWidth', 2);
        hold on;
        throttlePlot = plot(NaN, NaN, 'k:', 'LineWidth', 1);
        ylabel('Velocity (km/h) | Throttle %', 'FontSize', 10, 'FontName','Garamound');
        xlabel('Time (s)', 'FontSize', 10, 'FontName','Garamound');
        ylim([-5, 100])
        set(gca, 'FontSize', 15);
        grid on;

        subplot(3,7,12:14);
        deltaPlot = plot(NaN, NaN, 'b-', 'LineWidth', 2);
        hold on;
        steeringinPlot = plot(NaN, NaN, 'k:', 'LineWidth', 1);
        ylabel('Steering angle (rad)', 'FontSize', 10, 'FontName','Garamound');
        xlabel('Time (s)', 'FontSize', 10, 'FontName','Garamound');
        ylim([-1, 1])
        set(gca, 'FontSize', 15);
        grid on;

        subplot(3,7,19:21);
        posErrorPlot = plot(NaN, NaN, 'r-', 'LineWidth', 2);
        ylabel('Position error (m)', 'FontSize', 10, 'FontName','Garamound');
        xlabel('Time (s)', 'FontSize', 10, 'FontName','Garamound');
        %ylim([-0.2, 5])
        set(gca, 'FontSize', 15);
        grid on;
    end

    if isempty(refPathX)
        vehiclePathX = [];
        refPathX = [];
    end
    
    if isempty(refPathY)
        vehiclePathY = [];
        refPathY = [];
    end
    
    subplot(3,7,[1:3 8:10 15:17]);
    vehiclePathX(end+1) = x;
    vehiclePathY(end+1) = y;
    refPathX(end+1) = xref;
    refPathY(end+1) = yref;
    timeArray(end+1) = time;
    deltaArray(end+1) = delta;
    velocityArray(end+1) = velocity*3.6;
    throttleArray(end+1) = throttle;
    steeringinArray(end+1) = steeringin;

    tempError = Inf;

    if length(refPathX) > 150
        t100 = 0:99;

        X100 = refPathX(end-99:end);
        Y100 = refPathY(end-99:end);

        tq = 0:0.002:99;

        xq = interp1(t100, X100, tq, 'linear');
        yq = interp1(t100, Y100, tq, 'linear');

        for i = 1:45000
            itError = sqrt( (x - xq(end - (i)))^2 + (y - yq(end - (i)))^2 );
            if itError < tempError
                tempError = itError;
            end
        end
    end

    errorArray(end+1) = tempError;

    leftWheelVertices = [-wheelWidth/2, -wheelHeight/2;
                    wheelWidth/2, -wheelHeight/2;
                    wheelWidth/2, wheelHeight/2;
                    -wheelWidth/2, wheelHeight/2];

    rightWheelVertices = [-wheelWidth/2, -wheelHeight/2;
                    wheelWidth/2, -wheelHeight/2;
                    wheelWidth/2, wheelHeight/2;
                    -wheelWidth/2, wheelHeight/2];

    rearLeftWheelVertices = [-wheelWidth/2, -wheelHeight/2;
                    wheelWidth/2, -wheelHeight/2;
                    wheelWidth/2, wheelHeight/2;
                    -wheelWidth/2, wheelHeight/2];

    rearRightWheelVertices = [-wheelWidth/2, -wheelHeight/2;
                    wheelWidth/2, -wheelHeight/2;
                    wheelWidth/2, wheelHeight/2;
                    -wheelWidth/2, wheelHeight/2];

    lwVertices = [-lwWidth/2, -lwHeight/2;
                    lwWidth/2, -lwHeight/2;
                    lwWidth/2, lwHeight/2;
                    -lwWidth/2, lwHeight/2];
    
    R = [cos(psi), -sin(psi); sin(psi), cos(psi)];
    rotatedLW = (R * lwVertices')';
    fW = [cos(psi+delta), -sin(psi+delta); sin(psi+delta), cos(psi+delta)];
    rW = [cos(psi), -sin(psi); sin(psi), cos(psi)];
    rotatedLeftWheel = (fW * leftWheelVertices')';
    rotatedRightWheel = (fW * rightWheelVertices')';
    rotatedRearLeftWheel = (rW * rearLeftWheelVertices')';
    rotatedRearRightWheel = (rW * rearRightWheelVertices')';
    
    translatedLW = rotatedLW + [x, y];
    translatedLeftWheel = rotatedLeftWheel + [x + cos(psi + pi/2) + cos(psi), y + sin(psi + pi/2) + sin(psi)];
    translatedRightWheel = rotatedRightWheel + [x + cos(psi - pi/2) + cos(psi), y + sin(psi - pi/2) + sin(psi)];
    translatedRearLeftWheel = rotatedRearLeftWheel + [x + cos(psi + pi/2) - cos(psi), y + sin(psi + pi/2) - sin(psi)];
    translatedRearRightWheel = rotatedRearRightWheel + [x + cos(psi - pi/2) - cos(psi), y + sin(psi - pi/2) - sin(psi)];
    
    set(leftWheelPatch, 'XData', translatedLeftWheel(:,1), 'YData', translatedLeftWheel(:,2));
    set(rightWheelPatch, 'XData', translatedRightWheel(:,1), 'YData', translatedRightWheel(:,2));
    set(rearLeftWheelPatch, 'XData', translatedRearLeftWheel(:,1), 'YData', translatedRearLeftWheel(:,2));
    set(rearRightWheelPatch, 'XData', translatedRearRightWheel(:,1), 'YData', translatedRearRightWheel(:,2));
    set(lwPatch, 'XData', translatedLW(:,1), 'YData', translatedLW(:,2));
    set(pathPlot, 'XData', vehiclePathX, 'YData', vehiclePathY);
    set(refPlot, 'XData', refPathX, 'YData', refPathY);
    
    main_lim = 20;
    xlim([x-main_lim, x+main_lim]);
    if x - 15 < xmin
        xmin = x-15;
    end
    if x + 15 > xmax
        xmax = x+15;
    end
    ylim([y-main_lim, y+main_lim]);
    if y - 15 < ymin
        ymin = y-15;
    end
    if y + 15 > ymax
        ymax = y+15;
    end
    subplot(3,7,5:7);
    xlim([time-10, time+2]);
    set(velocityPlot, 'XData', timeArray,'YData', velocityArray);
    set(throttlePlot, 'XData', timeArray,'YData', throttleArray);

    subplot(3,7,12:14);
    xlim([time-10, time+2]);
    set(deltaPlot, 'XData', timeArray, 'YData', deltaArray);
    set(steeringinPlot, 'XData', timeArray,'YData', steeringinArray);
    
    subplot(3,7,19:21);
    xlim([time-10, time+2]);
    set(posErrorPlot, 'XData', timeArray, 'YData', errorArray);
    ylim([-0.1 , 1])
    drawnow
end

== matlab function LoneWolfSimulator/Subsystem5/Subsystem3/MATLAB Function ==
  data: alpha input; Fc output; kappa input; Bc parameter; Cc parameter; Dc parameter; Ec parameter; alpha_peak parameter; kappa_peak parameter
function Fc = fcn(alpha, kappa, Bc, Cc, Dc, Ec, alpha_peak, kappa_peak)

alpha_norm = alpha/alpha_peak;
kappa_norm = kappa/kappa_peak;

S = sqrt(alpha_norm^2+kappa_norm^2);

alpha_mod = S * alpha_peak;

Fc = alpha_norm/S * Dc*sin(Cc*atan(Bc*alpha_mod-Ec*(Bc*alpha_mod-atan(Bc*alpha_mod))));

== matlab function LoneWolfSimulator/Subsystem5/Subsystem2/MATLAB Function ==
  data: xd input; xdot output
function xdot = fcn(xd)

if xd == 0
    xdot = 0.001;
else
    xdot = xd;
end

== matlab function LoneWolfSimulator/Subsystem2/Longitudinal forces rear wheel/MATLAB Function ==
  data: xd input; xdot output
function xdot = fcn(xd)

if xd < 0.001
    xdot = 0.001;
else
    xdot = xd;
end

== matlab function LoneWolfSimulator/MATLAB Function10 ==
  data: xdot input; v output; ydot input
function v = fcn(xdot, ydot)

v = sqrt(xdot^2+ydot^2);

== matlab function LoneWolfSimulator/Subsystem5/Subsystem3/MATLAB Function11 ==
  data: Fl input; Fxf output; delta input
function Fxf = fcn(Fl, delta)

Fxf = Fl*cos(delta);

== matlab function LoneWolfSimulator/Subsystem2/Longitudinal forces rear wheel/Pacejka function ==
  data: Fx output; Bl parameter; Cl parameter; Dl parameter; El parameter; kappa_peak parameter; alpha_peak parameter; kappa input; alpha input
function Fx = fcn(Bl, Cl, Dl, El, kappa_peak, alpha_peak, kappa, alpha)

alpha_norm = alpha/alpha_peak;
kappa_norm = kappa/kappa_peak;

S = sqrt(alpha_norm^2+kappa_norm^2);

kappa_mod = S * alpha_peak;

Fx = kappa_norm/S * Dl*sin(Cl*atan(Bl*kappa_mod-El*(Bl*kappa_mod-atan(Bl*kappa_mod))));

== matlab function LoneWolfSimulator/Subsystem2/Longitudinal forces rear wheel/MATLAB Function16 ==
  data: T input; omegadot output; Fx input; omega input; wheelRadius parameter; Iw parameter; RRC parameter
function omegadot = fcn(T, Fx, omega, wheelRadius, Iw, RRC)

omegadot = (T - wheelRadius * Fx - RRC * omega)/Iw;

% 0.5 = Hjulets treghetsmoment
% 8 * omega motorbrems / rullemotstand
